simulink model "DC_motor_MRAC_d"  (R2015b)
settings: Solver=VariableStepAuto  StartTime=0.0  StopTime=20  RelTol=1e-3
undefined symbols (not defined in the file): Amd, Bmd, Cmd, Gammae, Gammau, Gammax, timestep
settings Model: Creator=mgreiff  LastModifiedBy=mgreiff

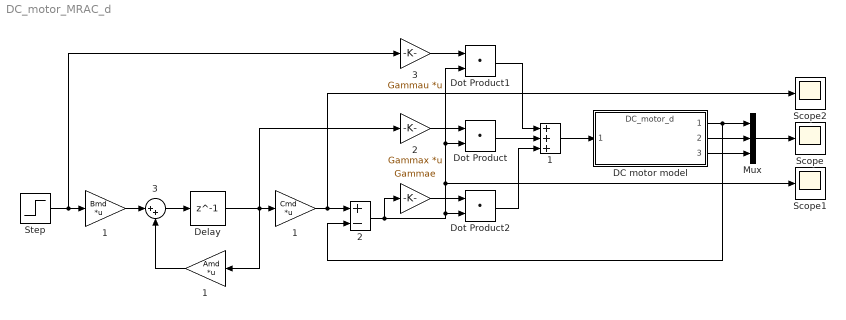
== system DC_motor_MRAC_d ==
  "   " : Gain  Gain=Gammae
  "       1" : Gain  Gain=Cmd  Multiplication=Matrix(K*u)
  "    1" : Gain  Gain=Amd  Multiplication=Matrix(K*u)
  "    2" : Gain  Gain=Gammax  Multiplication=Matrix(K*u)
  "    3" : Gain  Gain=Gammau  Multiplication=Matrix(K*u)
  "  1" : Gain  Gain=Bmd  Multiplication=Matrix(K*u)
  " 1" : Sum  Inputs=+++
  " 2" : Sum  Inputs=+-
  " 3" : Sum  Inputs=|++
  DC motor model : ModelReference  ModelNameDialog=DC_motor_d.slx  SimulationMode=Normal  ModelReferenceVersion=1.8  CopyOfModelName=DC_motor_d.slx
  Delay : Delay  DelayLength=1  SampleTime=timestep
  Dot Product : DotProduct  InputSameDT=on  OutDataTypeStr=Inherit: Inherit via internal rule
  Dot Product1 : DotProduct  InputSameDT=on  OutDataTypeStr=Inherit: Inherit via internal rule
  Dot Product2 : DotProduct  InputSameDT=on  OutDataTypeStr=Inherit: Inherit via internal rule
  Mux : Mux  Inputs=3
  Scope : Scope
  Scope1 : Scope
  Scope2 : Scope
  Step : Step  Time=0  SampleTime=0
  wires:
  " 3"/1 -> Delay/1
  "  1"/1 -> " 3"/1
  "    1"/1 -> " 3"/2
  Delay/1 -> "    1"/1, "       1"/1, "    2"/1
  "       1"/1 -> Scope2/1, " 2"/1
  " 2"/1 -> Dot Product2/2, Dot Product1/2, Dot Product/2, Scope1/1, "   "/1
  Step/1 -> "    3"/1, "  1"/1
  Dot Product/1 -> " 1"/2
  Dot Product1/1 -> " 1"/1
  " 1"/1 -> DC motor model/1
  "    2"/1 -> Dot Product/1
  "    3"/1 -> Dot Product1/1
  Dot Product2/1 -> " 1"/3
  "   "/1 -> Dot Product2/1
  DC motor model/3 -> Mux/3
  DC motor model/1 -> " 2"/2, Mux/1
  DC motor model/2 -> Mux/2
  Mux/1 -> Scope/1
